simulink model "twoLinkRobot"  (R2014b)
settings: Solver=ode45  StartTime=0.0  StopTime=10.0  RelTol=1e-3
undefined symbols (not defined in the file or in its folder): dof
libraries: cstblocks x2
settings Model: Creator=japerez  LastModifiedBy=japerez

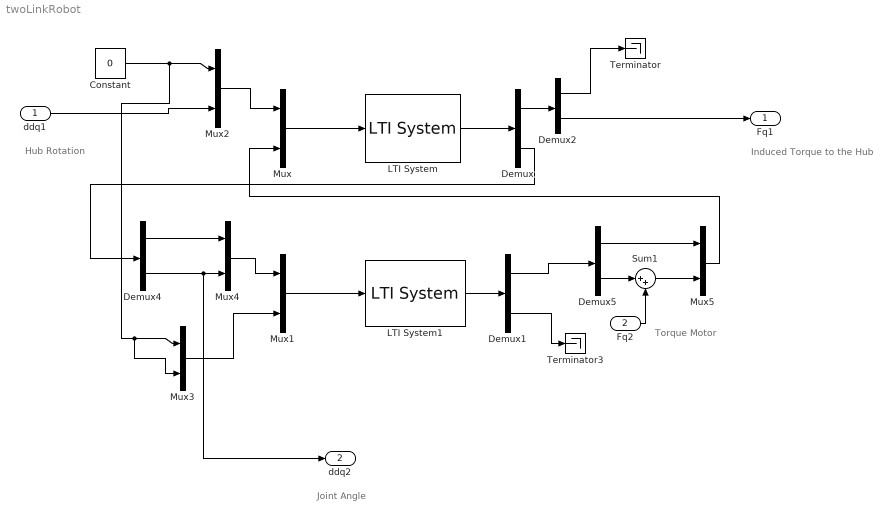
== system twoLinkRobot ==
  note: Induced Torque to the Hub
  note: Hub Rotation
  note: Joint Angle
  note: Torque Motor
  ddq1 : Inport
  Fq2 : Inport  Port=2
  Constant : Constant  Value=0
  Demux : Demux  Outputs=[dof dof]
  Demux1 : Demux  Outputs=[dof dof]
  Demux2 : Demux  Outputs=[ 1 1]
  Demux4 : Demux  Outputs=[1 1]
  Demux5 : Demux  Outputs=[ 1 1]
  LTI System : cstblocks/LTI System  sys=TITOPseg1  IC=[]
  LTI System1 : cstblocks/LTI System  sys=TITOPseg2  IC=[]
  Mux : Mux  Inputs=[dof dof]
  Mux1 : Mux  Inputs=[dof dof]
  Mux2 : Mux  Inputs=[1 1 ]
  Mux3 : Mux  Inputs=[ 1 1]
  Mux4 : Mux  Inputs=[1 1]
  Mux5 : Mux  Inputs=[1 1]
  Sum1 : Sum  Inputs=|++
  Terminator : Terminator
  Terminator3 : Terminator
  Fq1 : Outport
  ddq2 : Outport  Port=2
  wires:
  LTI System1/1 -> Demux1/1
  Demux1/1 -> Demux5/1
  Mux/1 -> LTI System/1
  LTI System/1 -> Demux/1
  Mux1/1 -> LTI System1/1
  Constant/1 -> Mux3/1, Mux3/2, Mux2/1
  Mux2/1 -> Mux/1
  Demux/1 -> Demux2/1
  Mux3/1 -> Mux1/2
  Demux2/1 -> Terminator/1
  Demux1/2 -> Terminator3/1
  Demux/2 -> Demux4/1
  Demux4/1 -> Mux4/1
  Mux4/1 -> Mux1/1
  Fq2/1 -> Sum1/2
  Demux5/1 -> Mux5/1
  Mux5/1 -> Mux/2
  ddq1/1 -> Mux2/2
  Demux5/2 -> Sum1/1
  Sum1/1 -> Mux5/2
  Demux2/2 -> Fq1/1
  Demux4/2 -> ddq2/1, Mux4/2
